simulink model "Model_nie_liniowy"  (R2017a)
settings: Solver=ode45  StartTime=0.0  StopTime=100  MaxStep=0.001  RelTol=1e-5  EnableMultiTasking=on
values from neighbouring files (symbols this model uses):
  L = lqr(A, B, Q, R)    [Linearyzacja_ramienia_robota.m]    (also in filtr_kalmana_Mateusz.m = (eye(4) - K*C_D)*B_D; sciaga.m = lqr(A,B,Q,R))
settings Model: Creator=kss  LastModifiedBy=Szwank
settings SolverCC: MaxConsecutiveZCs=100000  ZeroCrossControl=EnableAll  SolverResetMethod=Robust
settings OptimizationCC: LifeSpan=inf
settings DebuggingCC: SFUnexpectedBacktrackingDiag=warning  SFNoUnconditionalDefaultTransitionDiag=warning  SFExecutionAtInitializationDiag=none
settings GRTTargetCC: TargetLangStandard=C89/C90 (ANSI)  GeneratePreprocessorConditionals=Disable all
settings ConfigComp: CovMetricSettings=dw  CovHtmlReporting=on  CovSaveCumulativeToWorkspaceVar=on  CovSaveSingleToWorkspaceVar=on  CovExternalEMLEnable=off

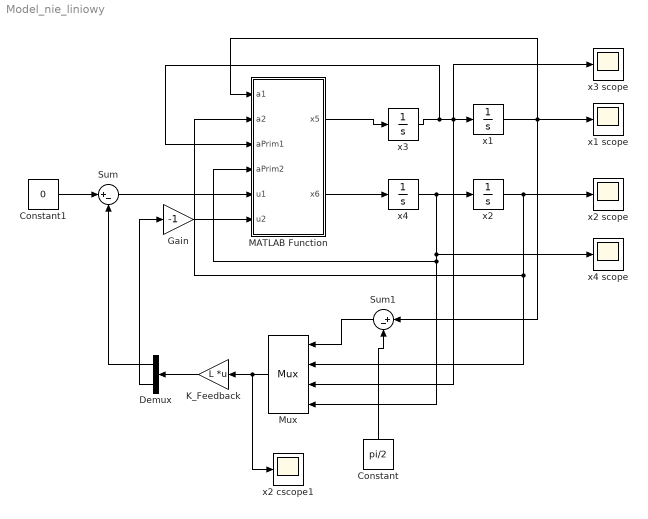
== system Model_nie_liniowy ==
  Constant : Constant  Value=pi/2
  Constant1 : Constant  Value=0
  Demux : Demux  Outputs=2
  Gain : Gain  Gain=-1
  K_Feedback : Gain  Gain=L  Multiplication=Matrix(K*u)
  MATLAB Function : MATLAB Function  TreatAsAtomicUnit=on
  Mux : Mux
      settings: DisplayOption=signals
  Sum : Sum  Inputs=|+-
  Sum1 : Sum  Inputs=|+-
  x1 : Integrator  InitialCondition=pi/2  AbsoluteTolerance=1e-5
  x1 scope : Scope
  x2 : Integrator  AbsoluteTolerance=1e-5
  x2 cscope1 : Scope
  x2 scope : Scope
  x3 : Integrator  AbsoluteTolerance=1e-5
  x3 scope : Scope
  x4 : Integrator  AbsoluteTolerance=1e-5
  x4 scope : Scope
  wires:
  MATLAB Function/1(x5) -> x3/1
  MATLAB Function/2(x6) -> x4/1
  x3/1 -> MATLAB Function/3(aPrim1), x3 scope/1, Mux/3, x1/1
  x4/1 -> x4 scope/1, Mux/4, MATLAB Function/4(aPrim2), x2/1
  x2/1 -> x2 scope/1, Mux/2, MATLAB Function/2(a2)
  x1/1 -> Sum1/1, x1 scope/1, MATLAB Function/1(a1)
  Mux/1 -> x2 cscope1/1, K_Feedback/1
  K_Feedback/1 -> Demux/1
  Demux/1 -> Sum/2
  Sum1/1 -> Mux/1
  Constant1/1 -> Sum/1
  Sum/1 -> MATLAB Function/5(u1)
  Demux/2 -> Gain/1
  Constant/1 -> Sum1/2
  Gain/1 -> MATLAB Function/6(u2)

== matlab function Model_nie_liniowy/MATLAB Function ==
  data: a1 input; a2 input; aPrim1 input; aPrim2 input; u1 input; u2 input; x5 output; x6 output
function [x5,x6] = fcn(a1,a2,aPrim1,aPrim2,u1,u2)
m1 = 2; m2 = 1; l1 = 1.5; l2 = 1; lc1 = l1/2; lc2 = l2/2; J1 = (m1*l1^2)/3; J2 = (m2*l2^2)/3; g = 9.81;
H11 = m1*lc1^2 + J1 + m2*(l1^2 + lc2^2 + 2*l1*l2*cos(a2)) + J2;
H12  = m2*l1*lc2*cos(a2) + m2*lc2^2 + J2;
H21 = H12;
H22 = m2*lc2^2 + J2;
h = m2*l1*lc2*sin(a2);
g1 = m1*lc1*g*cos(a1) + m2*g*(lc2*cos(a1+a2)+l1*cos(a1));
g2 = m2*lc2*g*cos(a1+a2);
H = [H11 H12; H21 H22];
H2 = inv(H);

J = [-h*aPrim2, -h*aPrim1-h*aPrim2; h*aPrim1,0];
M = [g1;g2];
U = [u1;u2];
%rozwikłanie 
Roz = -1*H2*J*[aPrim1; aPrim2] -1*H2*M + H2*U; 
x5 = Roz(1);
x6 = Roz(2);
% x5 = (200*T1 - 200*T2 + (2943*cos(x1 + 2*x2))/2 - (8829*cos(x1))/2 + 150*x3^2*sin(x2) + 150*x4^2*sin(x2) + 225*x3^2*sin(2*x2) - 23544*J2*cos(x1) - 600*T2*cos(x2) + 800*J2*T1 - 800*J2*T2 + 300*x3*x4*sin(x2) + 600*J2*x3^2*sin(x2) + 600*J2*x4^2*sin(x2) + 1200*J2*x3*x4*sin(x2))/(25*(8*J1 + 108*J2 - 9*cos(2*x2) + 32*J1*J2 + 18));
% x6 = -(400*T1 - 5800*T2 - 17658*cos(x1 - x2) + 2943*cos(x1 + 2*x2) + 8829*cos(x1 + x2) - 8829*cos(x1) + 4350*x3^2*sin(x2) + 300*x4^2*sin(x2) + 7848*J1*cos(x1 + x2) + 900*x3^2*sin(2*x2) + 450*x4^2*sin(2*x2) - 47088*J2*cos(x1) + 1200*T1*cos(x2) - 2400*T2*cos(x2) - 1600*J1*T2 + 1600*J2*T1 - 1600*J2*T2 + 600*x3*x4*sin(x2) + 1200*J1*x3^2*sin(x2) + 1200*J2*x3^2*sin(x2) + 1200*J2*x4^2*sin(x2) + 900*x3*x4*sin(2*x2) + 2400*J2*x3*x4*sin(x2))/(50*(8*J1 + 108*J2 - 9*cos(2*x2) + 32*J1*J2 + 18));

%y = u;
